simulink model "v_f_control_system"  (Simulink 8.9)
settings: Solver=ode23  StartTime=0.0  StopTime=5  RelTol=1e-3  EnableMultiTasking=on
undefined symbols (not defined in the file or in its folder): D1, Delta, DiscIntNeverNeededParam, Ts_Control, Ts_Power
libraries: powerlib x14, powerlib_meascontrol x9, simulink_extras x1, simulink x1
settings Model: Creator=Administrator  LastModifiedBy=Administrator
settings OptimizationCC: ExpressionDepthLimit=2147483647
settings DebuggingCC: SolverPrmCheckMsg=warning
settings GRTTargetCC: CombineOutputUpdateFcns=on  GRTInterface=off

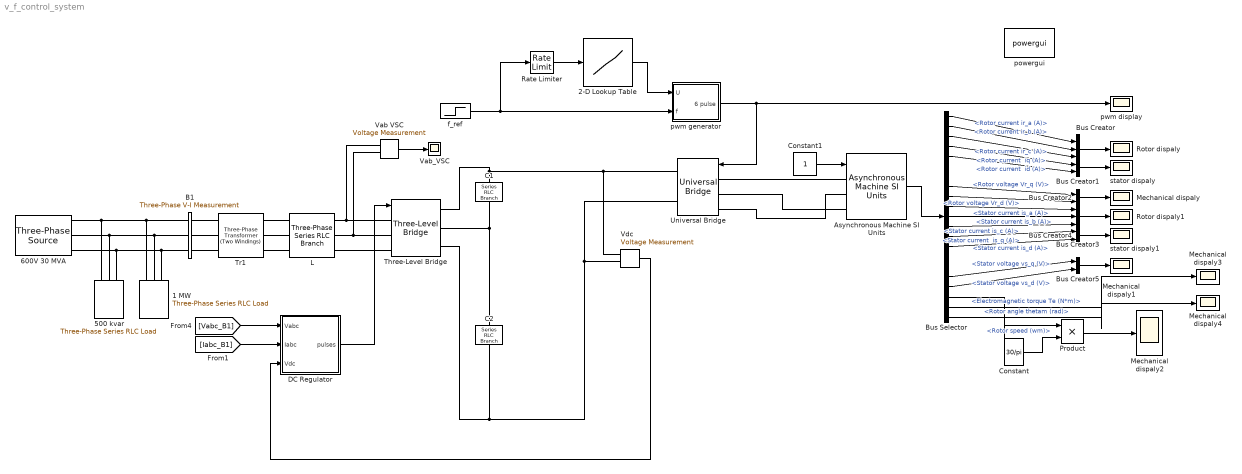
== system v_f_control_system ==
  1 MW : powerlib/Elements/Three-Phase Series RLC Load  LConnTagsString=A|B|C  Configuration=Y (grounded)  NominalVoltage=600  Vabc=[1e3 1e3 1e3]  Vabcp=[1e3 1e3 1e3]  NominalFrequency=60  UnbalancedPower=off  ActivePower=1e6  InductivePower=0  CapacitivePower=0  Pabc=[10e3 9e3 11e3]  QLabc=[100 90 110]  QCabc=[100 90 110]  Pabcp=[10e3 9e3 11e3]  QLabcp=[100 90 110]  QCabcp=[100 90 110]  Measurements=None  LoadType=constant Z
  2-D Lookup Table : Lookup_n-D  NumberOfTableDimensions=1  BreakpointsForDimension1=[0 5 25 50 100]  BreakpointsForDimension2=[1:3]  Table=[0.1 0.1 0.5 1 1]  RndMeth=Simplest  InputSameDT=on
  500 kvar : powerlib/Elements/Three-Phase Series RLC Load  LConnTagsString=A|B|C  Configuration=Y (grounded)  NominalVoltage=600  Vabc=[1e3 1e3 1e3]  Vabcp=[1e3 1e3 1e3]  NominalFrequency=60  UnbalancedPower=off  ActivePower=0.5e6/100  InductivePower=0  CapacitivePower=0.5e6  Pabc=[10e3 9e3 11e3]  QLabc=[100 90 110]  QCabc=[100 90 110]  Pabcp=[10e3 9e3 11e3]  QLabcp=[100 90 110]  QCabcp=[100 90 110]  Measurements=None  LoadType=constant Z
  600V 30 MVA : powerlib/Electrical Sources/Three-Phase Source  InternalConnection=Yg  VoltagePhases=off  Voltage=110  PhaseAngle=0  Voltage_phases=[25e3 25e3 25e3]/sqrt(3)  PhaseAngles_phases=[0 -120 +120]  Frequency=60  NonIdealSource=on  SpecifyImpedance=on  Resistance=0.724  Inductance=19.2e-3  ShortCircuitLevel=30e6  BaseVoltage=600  XRratio=10  BusType=swing  Pref=0  Qref=0  Prefabc=[10e3, 10e3, 10e3]  Qrefabc=[0, 0, 0]  Qmin=-inf  Qmax=inf
  Asynchronous Machine SI Units : powerlib/Machines/Asynchronous Machine SI Units  RotorType=Squirrel-cage  PresetModel=No  MechanicalLoad=Torque Tm  ShowDetailedParameters=on  ReferenceFrame=Rotor  Units=SI  MeasurementBus=off  NominalParameters=[ 2200, 380, 50 ]  Stator=[ 3.478 0.01254]  Rotor=[ 2.546 0.01226]  Cage1=[ 0.022 0.226/377]  Cage2=[ 0.022 0.226/377]  Lm=0.3329  Mechanical="[ 0.0131  0  2 ]"  PolePairs=2  InitialConditions=[1 0 0 0 0 0 0 0]  SimulateSaturation=off  Saturation=[14.03593122, 27.81365428, 53.79336849, 72.68890987, 97.98006896, 148.6815601, 215.7428561, 302.9841135, 420.4778367 ; 230, 322, 414, 460, 506, 552, 598, 644, 690]  LoadFlowParameters=1492000  TsPowergui=0  TsBlock=-1  IterativeModel=Forward Euler  IterativeDiscreteModel=Trapezoidal non iterative  Pmec=0
  B1 : powerlib/Measurements/Three-Phase V-I Measurement  VoltageMeasurement=phase-to-ground  SetLabelV=on  LabelV=Vabc_B1  Vpu=off  VpuLL=off  CurrentMeasurement=yes  SetLabelI=on  LabelI=Iabc_B1  Ipu=off  Pbase=100e6  Vbase=500e3  OutputType=Magnitude  PhasorSimulation=off  PSBequivalent=0
  Bus Creator : BusCreator  Inputs=3
  Bus Creator{1..2,4..5} (4 alike) : BusCreator  Inputs=2
  Bus Creator3 : BusCreator  Inputs=3
  Bus Selector : BusSelector  OutputSignals="Rotor measurements.Rotor current ir_a (A),Rotor measurements.Rotor current ir_b (A),Rotor measurements.Rotor current ir_c (A),Rotor measurements.Rotor current  iq (A),Rotor measurements.Rotor current  id (A),Rotor measurements.Rotor flux phir_q (V s),Rotor measurements.Rotor flux phir_d (V s),Rotor measurements.Rotor voltage Vr_q (V),Rotor measurements.Rotor voltage Vr_d (V),Stator measurements.Stator current is_a (A),Stator measurements.Stator current is_b (A),Stator measurements.Stator current is_c (A),Stator measurements.Stator current  is_q (A),Stator measurements.Stator current is_d (A),Stator measurements.Stator flux phis_q (V s),Stator measurements.Stator flux phis_d (V s),Stator measurements.Stator voltage vs_q (V),Stator measurements.Stator voltage vs_d (V),Mechanical.Rotor speed (wm),Mechanical.Electromagnetic torque Te (N*m),Mechanical.Rotor angle thetam (rad)"
  C1 : powerlib/Elements/Series RLC Branch  LConnTagsString=__new0  RConnTagsString=__new0  BranchType=C  Resistance=1.0  Inductance=1.0  SetiL0=off  InitialCurrent=0  Capacitance=0.1  Setx0=off  InitialVoltage=0  Measurements=None
  C2 : powerlib/Elements/Series RLC Branch  LConnTagsString=__new0  RConnTagsString=__new0  BranchType=C  Resistance=1.0  Inductance=1.0  SetiL0=off  InitialCurrent=0  Capacitance=0.1  Setx0=off  InitialVoltage=0  Measurements=None
  Constant : Constant  Value=30/pi
  Constant1 : Constant
  DC Regulator : Subsystem  mask(DC Voltage Regulator){Vdc_Ref=155.56}
      mask prompts: Vdc_Ref "DC voltage setpoint (V):"
  L : powerlib/Elements/Three-Phase Series RLC Branch  LConnTagsString=A|B|C  RConnTagsString=A|B|C  BranchType=RL  Resistance=0.1e-3  Inductance=20e-6  Capacitance=inf  Measurements=None
  Mechanical dispaly{,1..4} (5 alike) : Scope
  Product : Product
  Rate Limiter : RateLimiter  RisingSlewLimit=200  FallingSlewLimit=-200
  Rotor dispaly : Scope
  Rotor dispaly1 : Scope
  Three-Level Bridge : powerlib/Power Electronics/Three-Level Bridge  Arms=3  SnubberResistance=50  SbubberCapacitance=1e-6  Device=IGBT / Diodes  Ron=0.2e-3  ForwardVoltages="[  2 1 ]"  Measurements=All voltages and currents
      settings: SourceProductName=Simscape Power Systems  SourceProductBaseCode=PS
  Tr1 : powerlib/Elements/Three-Phase Transformer (Two Windings)  Winding1Connection=Yg  Winding2Connection=Delta (D1)  CoreType=Three single-phase transformers  SetSaturation=off  Hysteresis=off  DataFile='hysteresis'  SetInitialFlux=off  Measurements=None  UNITS=pu  NominalPower=[ 500e3 , 60 ]  Winding1=[ 110 , 0.04/30/2 , 0.04 ]  Winding2=[ 80 , 0.04/30/2 , 0.0 ]  Rm=500  Lm=500  L0=0.5  Saturation=[ 0,0 ; 0.0024,1.2 ; 1.0,1.52 ]  InitialFluxes=[ 0.8 , -0.8 , 0.7 ]  MoreParameters=off  BreakLoop=off  DataType=off  TransfoNumber=0
  Universal Bridge : powerlib/Power Electronics/Universal Bridge  Arms=3  SnubberResistance=1e5  SnubberCapacitance=inf  Device=IGBT / Diodes  Ron=1e-3  Lon=0  ForwardVoltages="[  0  0  ]"  ForwardVoltage=0  GTOparameters=[ 10e-6 , 20e-6 ]  IGBTparameters=[ 1e-6 , 2e-6 ]  Measurements=None  Measurements_2=None  converterType=Rectifier
  Vab VSC : powerlib/Measurements/Voltage Measurement  Tag=PoWeRsYsTeMmEaSuReMeNt  PhasorSimulation=off  OutputType=Magnitude  PSBequivalent=0
  Vab_VSC : Scope
  "Vdc " : powerlib/Measurements/Voltage Measurement  Tag=PoWeRsYsTeMmEaSuReMeNt  PhasorSimulation=off  OutputType=Magnitude  PSBequivalent=0
  f_ref : Step  Time=100  Before=33  After=33  SampleTime=0
  powergui : powerlib/powergui  Priority=1  SimulationMode=Discrete  SampleTime=1e-5  frequency=60  Iterations=50  frequencyindice=50  Pbase=100e6  ErrMax=1e-4  UnitsV=kV  UnitsW=MW  buscounter=0  FunctionMessages=off  echomessages=off  EnableUseOfTLC=off  CurrentSourceSwitches=off  DisableSnubberDevices=off  DisableRonSwitches=off  DisableVfSwitches=off  DisplayEquations=off  SolverType=Tustin  Interpol=off  ExternalGateDelay=off  methode=off  Ts=100  x0status=blocks  SPID=off  SwTol=0  HookPort=off  RestoreLinks=warning  ResistiveCurrentMeasurement=off  Frange=[0:2:500]  Ylog=off  Xlog=on  ShowGrid=off  save=off  variable=ZData  structure=0  ZoomFFT=off  StartTime=0.0  cycles=1  DisplayStyle=1  fundamental=60  FreqAxis=off  MaxFrequency=1000  frequencyindicesteady=1  RmsSteady=1  display=off
  pwm display : Scope
  pwm generator : Subsystem
  stator dispaly : Scope
  stator dispaly1 : Scope
  wires:
  pwm generator/1(6 pulse) -> Universal Bridge/1, pwm display/1
  f_ref/1 -> pwm generator/2(f), Rate Limiter/1
  Rate Limiter/1 -> 2-D Lookup Table/1
  2-D Lookup Table/1 -> pwm generator/1(U)
  Constant1/1 -> Asynchronous Machine SI Units/1
  Asynchronous Machine SI Units/1 -> Bus Selector/1
  Bus Selector/1 -> Bus Creator/1  "<Rotor current ir_a (A)>"
  Bus Selector/2 -> Bus Creator/2  "<Rotor current ir_b (A)>"
  Bus Selector/3 -> Bus Creator/3  "<Rotor current ir_c (A)>"
  Bus Creator/1 -> Rotor dispaly/1
  Bus Selector/4 -> Bus Creator1/1  "<Rotor current  iq (A)>"
  Bus Selector/5 -> Bus Creator1/2  "<Rotor current  id (A)>"
  Bus Selector/8 -> Bus Creator2/1  "<Rotor voltage Vr_q (V)>"
  Bus Selector/9 -> Bus Creator2/2  "<Rotor voltage Vr_d (V)>"
  Bus Creator1/1 -> stator dispaly/1
  Bus Creator2/1 -> Mechanical dispaly/1
  Bus Creator3/1 -> Rotor dispaly1/1
  Bus Creator4/1 -> stator dispaly1/1
  Bus Creator5/1 -> Mechanical dispaly1/1
  Bus Selector/10 -> Bus Creator3/1  "<Stator current is_a (A)>"
  Bus Selector/11 -> Bus Creator3/2  "<Stator current is_b (A)>"
  Bus Selector/12 -> Bus Creator3/3  "<Stator current is_c (A)>"
  Bus Selector/13 -> Bus Creator4/1  "<Stator current  is_q (A)>"
  Bus Selector/14 -> Bus Creator4/2  "<Stator current is_d (A)>"
  Bus Selector/17 -> Bus Creator5/1  "<Stator voltage vs_q (V)>"
  Bus Selector/18 -> Bus Creator5/2  "<Stator voltage vs_d (V)>"
  Bus Selector/20 -> Mechanical dispaly3/1  "<Electromagnetic torque Te (N*m)>"
  Bus Selector/21 -> Mechanical dispaly4/1  "<Rotor angle thetam (rad)>"
  Bus Selector/19 -> Product/1  "<Rotor speed (wm)>"
  Constant/1 -> Product/2
  Product/1 -> Mechanical dispaly2/1
  Vab VSC/1 -> Vab_VSC/1
  [Iabc_B1] -> DC Regulator/2(Iabc)
  "Vdc "/1 -> DC Regulator/3(Vdc)
  [Vabc_B1] -> DC Regulator/1(Vabc)
  DC Regulator/1(pulses) -> Three-Level Bridge/1
  connections:
  Universal Bridge/LConn1 -- Asynchronous Machine SI Units/LConn1
  C1/LConn1 -- Three-Level Bridge/RConn1 -- "Vdc "/LConn1 -- Universal Bridge/RConn1
  1 MW/LConn1 -- B1/LConn1 -- 500 kvar/LConn1 -- 600V 30 MVA/RConn1
  C1/RConn1 -- Three-Level Bridge/RConn2 -- C2/LConn1
  Three-Level Bridge/LConn2 -- Vab VSC/LConn2 -- L/RConn2
  1 MW/LConn3 -- B1/LConn3 -- 500 kvar/LConn3 -- 600V 30 MVA/RConn3
  1 MW/LConn2 -- B1/LConn2 -- 500 kvar/LConn2 -- 600V 30 MVA/RConn2
  Three-Level Bridge/LConn1 -- Vab VSC/LConn1 -- L/RConn1
  C2/RConn1 -- "Vdc "/LConn2 -- Universal Bridge/RConn2 -- Three-Level Bridge/RConn3
  Tr1/RConn1 -- L/LConn1
  B1/RConn2 -- Tr1/LConn2
  Tr1/RConn3 -- L/LConn3
  B1/RConn1 -- Tr1/LConn1
  B1/RConn3 -- Tr1/LConn3
  Tr1/RConn2 -- L/LConn2
  L/RConn3 -- Three-Level Bridge/LConn3
  Universal Bridge/LConn2 -- Asynchronous Machine SI Units/LConn3
  Universal Bridge/LConn3 -- Asynchronous Machine SI Units/LConn2

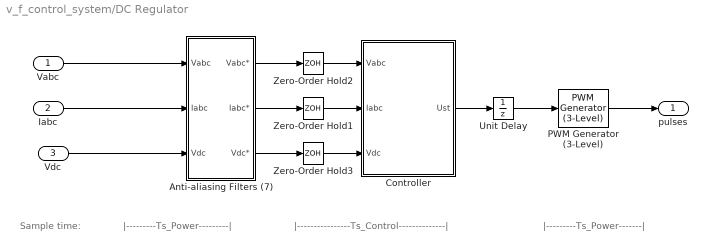
== system v_f_control_system/DC Regulator ==
  note: |----------------Ts_Control--------------|
  note: |---------Ts_Power---------|
  note: Sample time:
  note: |---------Ts_Power-------|
  Vabc : Inport  PortDimensions=3
  Iabc : Inport  Port=2  PortDimensions=3
  Vdc : Inport  Port=3  PortDimensions=1
  Anti-aliasing Filters (7) : Subsystem  mask(Anti-aliasing (2nd order lowpass)){Fc=750, Ts=Ts_Power}
      mask prompts: Fc "Cut-off frequency (Hz):"; Ts "Sample time:"
  Controller : Subsystem  mask(DC Regulator){Vdc_Ref=Vdc_Ref, Par_VdcReg=[0.015 1.6], Par_IReg=[0.3 20], Par_Nom=[600 500e3], Ts=Ts_Control}
      mask prompts: Vdc_Ref "DC Voltage setpoint (Volts)"; Par_VdcReg "Vdc Regulator Gains: [ Kp  Ki ]"; Par_IReg "Current Regulators Gain: [ Kp Ki Kd ]"; Par_Nom "Nominal Voltage and power: [ Vnom (volts rms L-L)  Pnom (VA) ]"; Ts "Time Step (s)"
      mask init:
      | Vnom=Par_Nom(1);
      | Pnom=Par_Nom(2);
      | Kp_I=Par_IReg(1);
      | Ki_I=Par_IReg(2);
      | Kp_Vdc=Par_VdcReg(1);
      | Ki_Vdc=Par_VdcReg(2);
  PWM Generator (3-Level) : powerlib_meascontrol/Pulse & Signal Generators/PWM Generator (3-Level)  ModulatorType=Three-phase bridge (12 pulses)  ModulatorMode=Unsynchronized  nF=27  Fc=27*60  ModulatingSignals=off  m=0.8  Freq=60  Phase=0  Ts=Ts_Power
      settings: SourceProductName=Simscape Power Systems  SourceProductBaseCode=PS
  Unit Delay : UnitDelay  SampleTime=Ts_Control
  Zero-Order Hold1 : ZeroOrderHold  SampleTime=Ts_Control
  Zero-Order Hold2 : ZeroOrderHold  SampleTime=Ts_Control
  Zero-Order Hold3 : ZeroOrderHold  SampleTime=Ts_Control
  pulses : Outport
  wires:
  PWM Generator (3-Level)/1 -> pulses/1
  Unit Delay/1 -> PWM Generator (3-Level)/1
  Controller/1(Ust) -> Unit Delay/1
  Anti-aliasing Filters (7)/1(" Vabc*") -> Zero-Order Hold2/1
  Anti-aliasing Filters (7)/2(Iabc*) -> Zero-Order Hold1/1
  Anti-aliasing Filters (7)/3(" Vdc*") -> Zero-Order Hold3/1
  Zero-Order Hold3/1 -> Controller/3(Vdc)
  Zero-Order Hold1/1 -> Controller/2(Iabc)
  Zero-Order Hold2/1 -> Controller/1(Vabc)
  Vdc/1 -> Anti-aliasing Filters (7)/3("Vdc ")
  Iabc/1 -> Anti-aliasing Filters (7)/2("Iabc ")
  Vabc/1 -> Anti-aliasing Filters (7)/1(Vabc)

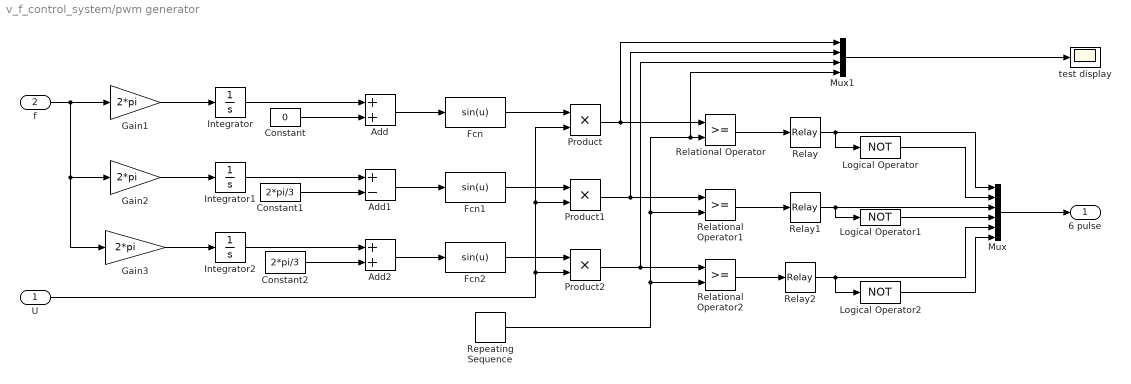
== system v_f_control_system/pwm generator ==
  U : Inport
  f : Inport  Port=2
  Add : Sum
  Add1 : Sum  Inputs=+-
  Add2 : Sum
  Constant : Constant  Value=0
  Constant1 : Constant  Value=2*pi/3
  Constant2 : Constant  Value=2*pi/3
  Fcn : Fcn  Expr=sin(u)
  Fcn1 : Fcn  Expr=sin(u)
  Fcn2 : Fcn  Expr=sin(u)
  Gain1 : Gain  Gain=2*pi
  Gain2 : Gain  Gain=2*pi
  Gain3 : Gain  Gain=2*pi
  Integrator : Integrator
  Integrator1 : Integrator
  Integrator2 : Integrator
  Logical Operator : Logic  Operator=NOT  AllPortsSameDT=off  OutDataTypeStr=boolean
  Logical Operator1 : Logic  Operator=NOT  AllPortsSameDT=off  OutDataTypeStr=boolean
  Logical Operator2 : Logic  Operator=NOT  AllPortsSameDT=off  OutDataTypeStr=boolean
  Mux : Mux  Inputs=6
  Mux1 : Mux
  Product : Product  RndMeth=Zero
  Product1 : Product  RndMeth=Zero
  Product2 : Product  RndMeth=Zero
  Relational Operator : RelationalOperator  OutDataTypeStr=boolean  RndMeth=Nearest
  Relational Operator1 : RelationalOperator  OutDataTypeStr=boolean  RndMeth=Nearest
  Relational Operator2 : RelationalOperator  OutDataTypeStr=boolean  RndMeth=Nearest
  Relay : Relay
  Relay1 : Relay
  Relay2 : Relay
  Repeating Sequence : simulink/Sources/Repeating Sequence  rep_seq_t=[0 0.5/3000 1/3000]  rep_seq_y=[-1 1 -1]
  test display : Scope
  6 pulse : Outport
  wires:
  f/1 -> Gain1/1, Gain3/1, Gain2/1
  Gain1/1 -> Integrator/1
  Gain2/1 -> Integrator1/1
  Gain3/1 -> Integrator2/1
  Integrator/1 -> Add/1
  Integrator1/1 -> Add1/1
  Integrator2/1 -> Add2/1
  Constant/1 -> Add/2
  Constant1/1 -> Add1/2
  Constant2/1 -> Add2/2
  Add/1 -> Fcn/1
  Add1/1 -> Fcn1/1
  Add2/1 -> Fcn2/1
  Repeating Sequence/1 -> Relational Operator2/2, Relational Operator1/2, Relational Operator/2, Mux1/4
  Relational Operator/1 -> Relay/1
  Relational Operator1/1 -> Relay1/1
  Relational Operator2/1 -> Relay2/1
  Mux/1 -> 6 pulse/1
  Fcn/1 -> Product/1
  Fcn2/1 -> Product2/1
  Fcn1/1 -> Product1/1
  U/1 -> Product1/2, Product/2, Product2/2
  Product/1 -> Relational Operator/1, Mux1/1
  Product2/1 -> Relational Operator2/1, Mux1/3
  Product1/1 -> Relational Operator1/1, Mux1/2
  Relay/1 -> Mux/1, Logical Operator/1
  Logical Operator/1 -> Mux/2
  Relay1/1 -> Mux/3, Logical Operator1/1
  Logical Operator1/1 -> Mux/4
  Relay2/1 -> Mux/5, Logical Operator2/1
  Logical Operator2/1 -> Mux/6
  Mux1/1 -> test display/1

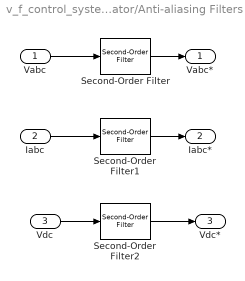
== system v_f_control_system/DC Regulator/Anti-aliasing Filters (7) ==
  Vabc : Inport  PortDimensions=3
  "Iabc " : Inport  Port=2  PortDimensions=3
  "Vdc " : Inport  Port=3  PortDimensions=1
  Second-Order Filter : powerlib_meascontrol/Filters/Second-Order Filter  FilterType=Lowpass  Fo=Fc  Zeta=0.707  Ts=Ts  Initialize=off  Vac_Init="[0,  0,  60]"  Vdc_Init=0  PlotResponse=off  FreqRange=[0, 500, 1]
      settings: SourceProductName=Simscape Power Systems  SourceProductBaseCode=PS
  Second-Order Filter1 : powerlib_meascontrol/Filters/Second-Order Filter  FilterType=Lowpass  Fo=Fc  Zeta=0.707  Ts=Ts  Initialize=off  Vac_Init="[0,  0,  60]"  Vdc_Init=0  PlotResponse=off  FreqRange=[0, 500, 1]
      settings: SourceProductName=Simscape Power Systems  SourceProductBaseCode=PS
  Second-Order Filter2 : powerlib_meascontrol/Filters/Second-Order Filter  FilterType=Lowpass  Fo=Fc  Zeta=0.707  Ts=Ts  Initialize=off  Vac_Init="[0,  0,  60]"  Vdc_Init=0  PlotResponse=off  FreqRange=[0, 500, 1]
      settings: SourceProductName=Simscape Power Systems  SourceProductBaseCode=PS
  " Vabc*" : Outport
  Iabc* : Outport  Port=2
  " Vdc*" : Outport  Port=3
  wires:
  Second-Order Filter2/1 -> " Vdc*"/1
  "Vdc "/1 -> Second-Order Filter2/1
  Vabc/1 -> Second-Order Filter/1
  Second-Order Filter/1 -> " Vabc*"/1
  "Iabc "/1 -> Second-Order Filter1/1
  Second-Order Filter1/1 -> Iabc*/1

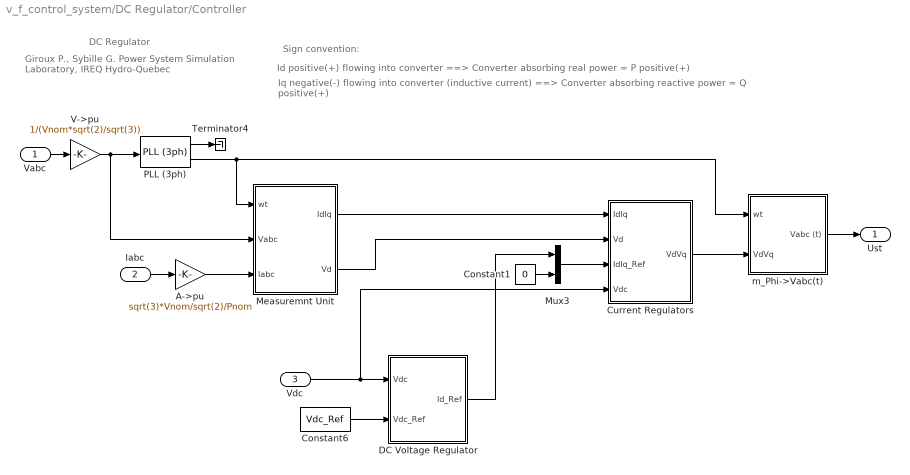
== system v_f_control_system/DC Regulator/Controller ==
  note: DC Regulator
  note: Giroux P., Sybille G.
      | Power System Simulation Laboratory, IREQ
      | Hydro-Quebec
  note: Iq negative(-) flowing into converter (inductive current) ==> Converter absorbing reactive power = Q positive(+)
  note: Sign convention:
  note: Id positive(+) flowing into converter ==> Converter absorbing real power = P positive(+)
  Vabc : Inport  PortDimensions=3
  Iabc : Inport  Port=2  PortDimensions=3
  Vdc : Inport  Port=3  PortDimensions=1
  A->pu : Gain  Gain=sqrt(3)*Vnom/sqrt(2)/Pnom  SaturateOnIntegerOverflow=on  OutDataTypeStr=Inherit: Same as input  ParamDataTypeStr=Inherit: Same as input
  Constant1 : Constant  Value=0
  Constant6 : Constant  Value=Vdc_Ref
  Current Regulators : Subsystem  mask(Current Regulators){Kp=Kp_I, Ki=Ki_I, Kd=0, TcD=0.2e-3, Par_Limits=[12 -12], Init=0, Ts=Ts}
      mask prompts: Kp "Proportional gain (Kp):"; Ki "Integral gain (Ki):"; Kd "Derivative gain (Kd):"; TcD "Time constant for derivative (s):"; Par_Limits "Output limits: [ Upper   Lower ]"; Init "Output initial value:"; Ts "Sample time:"
      mask help:
      | Sign convention:
      | Id positive(+) flowing into converter ==> Converter absorbing real power = P positive(+)
      | Iq negative(-) flowing into converter (inductive current) ==> Converter absorbing reactive power = Q positive(+)
  DC Voltage Regulator : Subsystem  mask(DC Voltage regulator){Kp=Kp_Vdc, Ki=Ki_Vdc, Ts=Ts}
      mask prompts: Kp "Proportional gain (Kp):"; Ki "Integral gain(Ki)"; Ts "Sample time:"
  Measuremnt Unit : Subsystem
  Mux3 : Mux  Inputs=2
  PLL (3ph) : powerlib_meascontrol/PLL/PLL (3ph)  Fmin=45  Par_Init=[-45 60]  ParK=[60 1400]  TcD=1e-4  MaxRateChangeFreq=12  FilterCutOffFreq=25  Ts=Ts  AGC=off
  Terminator4 : Terminator
  V->pu : Gain  Gain=1/(Vnom*sqrt(2)/sqrt(3))  SaturateOnIntegerOverflow=on  OutDataTypeStr=Inherit: Same as input  ParamDataTypeStr=Inherit: Same as input
  m_Phi->Vabc(t) : Subsystem
  Ust : Outport
  wires:
  m_Phi->Vabc(t)/1(Vabc (t)) -> Ust/1
  PLL (3ph)/2 -> m_Phi->Vabc(t)/1(wt), Measuremnt Unit/1(wt)
  Current Regulators/1(VdVq) -> m_Phi->Vabc(t)/2(VdVq)
  DC Voltage Regulator/1(Id_Ref) -> Mux3/1
  Constant1/1 -> Mux3/2
  Mux3/1 -> Current Regulators/3(IdIq_Ref)
  Measuremnt Unit/2(Vd) -> Current Regulators/2(Vd)
  Measuremnt Unit/1(IdIq) -> Current Regulators/1(IdIq)
  Iabc/1 -> A->pu/1
  PLL (3ph)/1 -> Terminator4/1
  Vdc/1 -> Current Regulators/4(Vdc), DC Voltage Regulator/1(Vdc)
  Constant6/1 -> DC Voltage Regulator/2(Vdc_Ref)
  Vabc/1 -> V->pu/1
  V->pu/1 -> PLL (3ph)/1, Measuremnt Unit/2(Vabc)
  A->pu/1 -> Measuremnt Unit/3(Iabc)

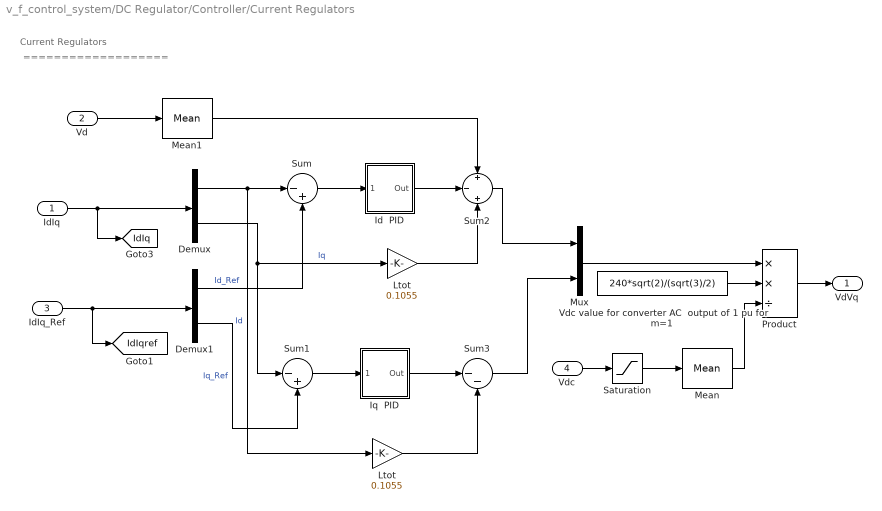
== system v_f_control_system/DC Regulator/Controller/Current Regulators ==
  note: ===================
  note: Current Regulators
  IdIq : Inport  PortDimensions=2
  Vd : Inport  Port=2
  IdIq_Ref : Inport  Port=3  PortDimensions=2
  Vdc : Inport  Port=4
  " Ltot" : Gain  Gain=0.1055  SaturateOnIntegerOverflow=on  OutDataTypeStr=Inherit: Same as input  ParamDataTypeStr=Inherit: Same as input
  Demux : Demux  Outputs=2
  Demux1 : Demux  Outputs=2
  Id  PID : Subsystem  DialogController=POWERSYS.PowerSysDialog  mask(Discrete PID Controller){Kp=Kp, Ki=Ki, Kd=Kd, TcD=TcD, Par_Limits=Par_Limits, Init=Init, Ts=Ts}
      mask prompts: Kp "Proportional gain (Kp):"; Ki "Integral gain (Ki):"; Kd "Derivative gain (Kd):"; TcD "Time constant for derivative (s):"; Par_Limits "Output limits: [ Upper   Lower ]"; Init "Output initial value:"; Ts "Sample time:"
      mask help: This block implements a discrete PID controller.
      mask init:
      | UpperLimit=Par_Limits(1);
      | LowerLimit=Par_Limits(2);
      | power_initmask();
      mask Display: disp('PID');
  Iq  PID : Subsystem  DialogController=POWERSYS.PowerSysDialog  mask(Discrete PID Controller){Kp=Kp, Ki=Ki, Kd=Kd, TcD=TcD, Par_Limits=Par_Limits, Init=Init, Ts=Ts}
      mask prompts: Kp "Proportional gain (Kp):"; Ki "Integral gain (Ki):"; Kd "Derivative gain (Kd):"; TcD "Time constant for derivative (s):"; Par_Limits "Output limits: [ Upper   Lower ]"; Init "Output initial value:"; Ts "Sample time:"
      mask help: This block implements a discrete PID controller.
      mask init:
      | UpperLimit=Par_Limits(1);
      | LowerLimit=Par_Limits(2);
      | power_initmask();
      mask Display: disp('PID');
  "Ltot " : Gain  Gain=0.1055  SaturateOnIntegerOverflow=on  OutDataTypeStr=Inherit: Same as input  ParamDataTypeStr=Inherit: Same as input
  Mean : powerlib_meascontrol/Measurements/Mean  Freq=60  Vinit=500  Ts=Ts
  Mean1 : powerlib_meascontrol/Measurements/Mean  Freq=60  Vinit=1.007  Ts=Ts
  Mux : Mux  Inputs=2
  Product : Product  Inputs=**/  SaturateOnIntegerOverflow=on  InputSameDT=on  OutDataTypeStr=Inherit: Same as first input
  Saturation : Saturate  UpperLimit=10000  LowerLimit=10
  Sum : Sum  Inputs=|-+  SaturateOnIntegerOverflow=on  InputSameDT=on  OutDataTypeStr=Inherit: Same as first input
  Sum1 : Sum  Inputs=|-+  SaturateOnIntegerOverflow=on  InputSameDT=on  OutDataTypeStr=Inherit: Same as first input
  Sum2 : Sum  Inputs=+|-|+  SaturateOnIntegerOverflow=on  InputSameDT=on  OutDataTypeStr=Inherit: Same as first input
  Sum3 : Sum  Inputs=|--  SaturateOnIntegerOverflow=on  InputSameDT=on  OutDataTypeStr=Inherit: Same as first input
  Vdc value for converter AC  output of 1 pu for m=1 : Constant  Value=240*sqrt(2)/(sqrt(3)/2)
  VdVq : Outport
  tag scope: IdIq=global, IdIqref=global
  wires:
  Sum3/1 -> Mux/2
  Vdc/1 -> Saturation/1
  Mean/1 -> Product/3
  Vdc value for converter AC  output of 1 pu for m=1/1 -> Product/2
  Saturation/1 -> Mean/1
  Mean1/1 -> Sum2/1
  Product/1 -> VdVq/1
  IdIq_Ref/1 -> [IdIqref], Demux1/1
  Mux/1 -> Product/1
  Sum/1 -> Id  PID/1(Error)
  Demux1/2 -> Sum1/2  "Iq_Ref"
  Sum1/1 -> Iq  PID/1(Error)
  Demux/2 -> Sum1/1, "Ltot "/1  "Iq"
  Demux1/1 -> Sum/2  "Id_Ref"
  Demux/1 -> " Ltot"/1, Sum/1  "Id"
  IdIq/1 -> [IdIq], Demux/1
  Id  PID/1(Out) -> Sum2/2
  Sum2/1 -> Mux/1
  Iq  PID/1(Out) -> Sum3/1
  "Ltot "/1 -> Sum2/3
  " Ltot"/1 -> Sum3/2
  Vd/1 -> Mean1/1

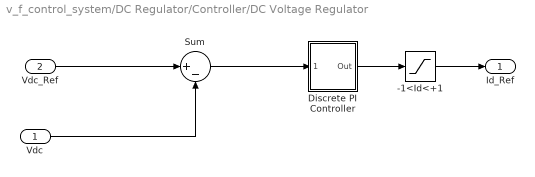
== system v_f_control_system/DC Regulator/Controller/DC Voltage Regulator ==
  Vdc : Inport
  Vdc_Ref : Inport  Port=2
  -1<Id<+1 : Saturate  UpperLimit=1.2  LowerLimit=-1.2
  Discrete PI Controller : Subsystem  DialogController=POWERSYS.PowerSysDialog  mask(Discrete PI Controller){Kp=Kp, Ki=Ki, Par_Limits=[1.2 -1.2], Init=0, Ts=Ts}
      mask prompts: Kp "Proportional gain (Kp):"; Ki "Integral gain (Ki):"; Par_Limits "Output limits: [ Upper   Lower ]"; Init "Output initial value:"; Ts "Sample time:"
      mask help: This block implements a discrete PI controller.
      mask init:
      | UpperLimit=Par_Limits(1);
      | LowerLimit=Par_Limits(2);
      | power_initmask();
      mask Display: disp('PI');
  Sum : Sum  Inputs=|+-  SaturateOnIntegerOverflow=on  InputSameDT=on  OutDataTypeStr=Inherit: Same as first input
  Id_Ref : Outport  InitialOutput=0
  wires:
  Sum/1 -> Discrete PI Controller/1(Error)
  Vdc/1 -> Sum/2
  Discrete PI Controller/1(Out) -> -1<Id<+1/1
  -1<Id<+1/1 -> Id_Ref/1
  Vdc_Ref/1 -> Sum/1

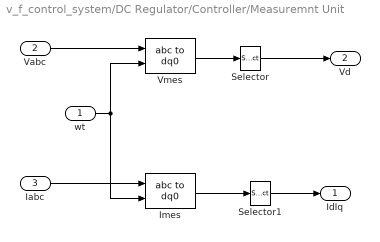
== system v_f_control_system/DC Regulator/Controller/Measuremnt Unit ==
  wt : Inport
  Vabc : Inport  Port=2
  Iabc : Inport  Port=3
  Imes : powerlib_meascontrol/Transformations/abc to dq0  Alignment=90 degrees behind phase A axis
  Selector : Selector  InputPortWidth=3  IndexOptions=Index vector (dialog)  Indices=1  OutputSizes=1
  Selector1 : Selector  InputPortWidth=3  IndexOptions=Index vector (dialog)  Indices=[1 2]  OutputSizes=1
  Vmes : powerlib_meascontrol/Transformations/abc to dq0  Alignment=90 degrees behind phase A axis
  IdIq : Outport
  Vd : Outport  Port=2
  wires:
  Selector/1 -> Vd/1
  Imes/1 -> Selector1/1
  Iabc/1 -> Imes/1
  wt/1 -> Imes/2, Vmes/2
  Vmes/1 -> Selector/1
  Vabc/1 -> Vmes/1
  Selector1/1 -> IdIq/1

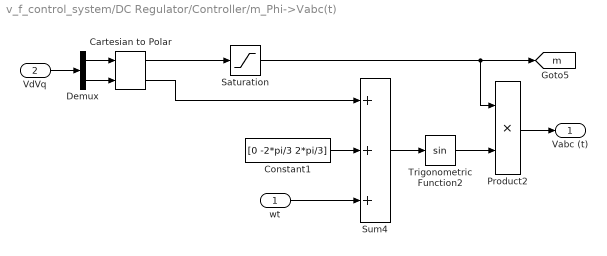
== system v_f_control_system/DC Regulator/Controller/m_Phi->Vabc(t) ==
  wt : Inport
  VdVq : Inport  Port=2
  Cartesian to Polar : simulink_extras/Transformations/Cartesian to Polar
      settings: SourceProductName=Simulink Extras
  Constant1 : Constant  Value=[0 -2*pi/3 2*pi/3]
  Demux : Demux  Outputs=2
  Product2 : Product  SaturateOnIntegerOverflow=on  InputSameDT=on  OutDataTypeStr=Inherit: Same as first input
  Saturation : Saturate  UpperLimit=1  LowerLimit=0
  Sum4 : Sum  Inputs=+++  SaturateOnIntegerOverflow=on  InputSameDT=on  OutDataTypeStr=Inherit: Same as first input
  Trigonometric Function2 : Trigonometry
  Vabc (t) : Outport
  tag scope: m=global
  wires:
  Saturation/1 -> [m], Product2/1
  Cartesian to Polar/1 -> Saturation/1
  Trigonometric Function2/1 -> Product2/2
  Sum4/1 -> Trigonometric Function2/1
  Cartesian to Polar/2 -> Sum4/1
  Demux/2 -> Cartesian to Polar/2
  Demux/1 -> Cartesian to Polar/1
  VdVq/1 -> Demux/1
  wt/1 -> Sum4/3
  Product2/1 -> Vabc (t)/1
  Constant1/1 -> Sum4/2

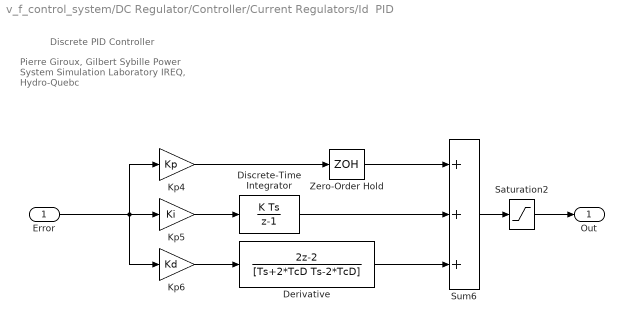
== system v_f_control_system/DC Regulator/Controller/Current Regulators/Id  PID ==
  note: Pierre Giroux, Gilbert Sybille
      | Power System Simulation Laboratory
      | IREQ, Hydro-Quebc
  note: Discrete PID Controller
  Error : Inport  SampleTime=Ts
  "Derivative " : DiscreteTransferFcn  Numerator=[2 -2]  Denominator=[Ts+2*TcD Ts-2*TcD]  SampleTime=Ts
  Discrete-Time Integrator : DiscreteIntegrator  InitialCondition=Init  SampleTime=Ts  LimitOutput=on  UpperSaturationLimit=UpperLimit  LowerSaturationLimit=LowerLimit  ICPrevOutput=DiscIntNeverNeededParam  ICPrevScaledInput=DiscIntNeverNeededParam
  Kp4 : Gain  Gain=Kp  SampleTime=Ts  SaturateOnIntegerOverflow=on  OutDataTypeStr=Inherit: Same as input  ParamDataTypeStr=Inherit: Same as input
  Kp5 : Gain  Gain=Ki  SampleTime=Ts  SaturateOnIntegerOverflow=on  OutDataTypeStr=Inherit: Same as input  ParamDataTypeStr=Inherit: Same as input
  Kp6 : Gain  Gain=Kd  SampleTime=Ts  SaturateOnIntegerOverflow=on  OutDataTypeStr=Inherit: Same as input  ParamDataTypeStr=Inherit: Same as input
  Saturation2 : Saturate  UpperLimit=UpperLimit  LowerLimit=LowerLimit  SampleTime=Ts
  Sum6 : Sum  Inputs=+++  SampleTime=Ts  SaturateOnIntegerOverflow=on  InputSameDT=on  OutDataTypeStr=Inherit: Same as first input
  Zero-Order Hold : ZeroOrderHold  SampleTime=Ts
  Out : Outport  SampleTime=Ts  InitialOutput=0
  wires:
  Saturation2/1 -> Out/1
  Error/1 -> Kp4/1, Kp5/1, Kp6/1
  Sum6/1 -> Saturation2/1
  Kp5/1 -> Discrete-Time Integrator/1
  Kp6/1 -> "Derivative "/1
  Kp4/1 -> Zero-Order Hold/1
  Discrete-Time Integrator/1 -> Sum6/2
  "Derivative "/1 -> Sum6/3
  Zero-Order Hold/1 -> Sum6/1

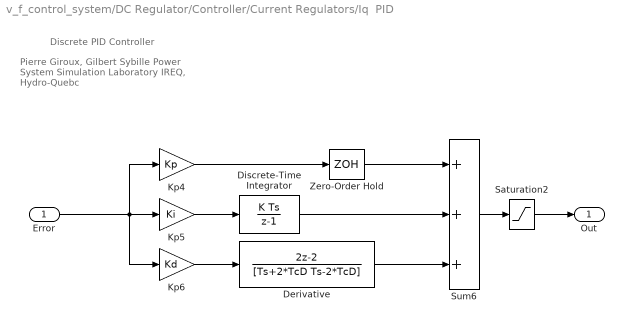
== system v_f_control_system/DC Regulator/Controller/Current Regulators/Iq  PID ==
  note: Pierre Giroux, Gilbert Sybille
      | Power System Simulation Laboratory
      | IREQ, Hydro-Quebc
  note: Discrete PID Controller
  Error : Inport  SampleTime=Ts
  "Derivative " : DiscreteTransferFcn  Numerator=[2 -2]  Denominator=[Ts+2*TcD Ts-2*TcD]  SampleTime=Ts
  Discrete-Time Integrator : DiscreteIntegrator  InitialCondition=Init  SampleTime=Ts  LimitOutput=on  UpperSaturationLimit=UpperLimit  LowerSaturationLimit=LowerLimit  ICPrevOutput=DiscIntNeverNeededParam  ICPrevScaledInput=DiscIntNeverNeededParam
  Kp4 : Gain  Gain=Kp  SampleTime=Ts  SaturateOnIntegerOverflow=on  OutDataTypeStr=Inherit: Same as input  ParamDataTypeStr=Inherit: Same as input
  Kp5 : Gain  Gain=Ki  SampleTime=Ts  SaturateOnIntegerOverflow=on  OutDataTypeStr=Inherit: Same as input  ParamDataTypeStr=Inherit: Same as input
  Kp6 : Gain  Gain=Kd  SampleTime=Ts  SaturateOnIntegerOverflow=on  OutDataTypeStr=Inherit: Same as input  ParamDataTypeStr=Inherit: Same as input
  Saturation2 : Saturate  UpperLimit=UpperLimit  LowerLimit=LowerLimit  SampleTime=Ts
  Sum6 : Sum  Inputs=+++  SampleTime=Ts  SaturateOnIntegerOverflow=on  InputSameDT=on  OutDataTypeStr=Inherit: Same as first input
  Zero-Order Hold : ZeroOrderHold  SampleTime=Ts
  Out : Outport  SampleTime=Ts  InitialOutput=0
  wires:
  Saturation2/1 -> Out/1
  Error/1 -> Kp4/1, Kp5/1, Kp6/1
  Sum6/1 -> Saturation2/1
  Kp5/1 -> Discrete-Time Integrator/1
  Kp6/1 -> "Derivative "/1
  Kp4/1 -> Zero-Order Hold/1
  Discrete-Time Integrator/1 -> Sum6/2
  "Derivative "/1 -> Sum6/3
  Zero-Order Hold/1 -> Sum6/1

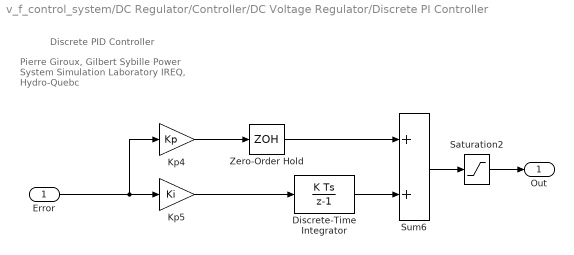
== system v_f_control_system/DC Regulator/Controller/DC Voltage Regulator/Discrete PI Controller ==
  note: Discrete PID Controller
  note: Pierre Giroux, Gilbert Sybille
      | Power System Simulation Laboratory
      | IREQ, Hydro-Quebc
  Error : Inport  SampleTime=Ts
  Discrete-Time Integrator : DiscreteIntegrator  InitialCondition=Init  SampleTime=Ts  LimitOutput=on  UpperSaturationLimit=UpperLimit  LowerSaturationLimit=LowerLimit  ICPrevOutput=DiscIntNeverNeededParam  ICPrevScaledInput=DiscIntNeverNeededParam
  Kp4 : Gain  Gain=Kp  SampleTime=Ts  SaturateOnIntegerOverflow=on  OutDataTypeStr=Inherit: Same as input  ParamDataTypeStr=Inherit: Same as input
  Kp5 : Gain  Gain=Ki  SampleTime=Ts  SaturateOnIntegerOverflow=on  OutDataTypeStr=Inherit: Same as input  ParamDataTypeStr=Inherit: Same as input
  Saturation2 : Saturate  UpperLimit=UpperLimit  LowerLimit=LowerLimit  SampleTime=Ts
  Sum6 : Sum  SampleTime=Ts  SaturateOnIntegerOverflow=on  InputSameDT=on  OutDataTypeStr=Inherit: Same as first input
  Zero-Order Hold : ZeroOrderHold  SampleTime=Ts
  Out : Outport  SampleTime=Ts  InitialOutput=0
  wires:
  Zero-Order Hold/1 -> Sum6/1
  Saturation2/1 -> Out/1
  Discrete-Time Integrator/1 -> Sum6/2
  Kp4/1 -> Zero-Order Hold/1
  Kp5/1 -> Discrete-Time Integrator/1
  Sum6/1 -> Saturation2/1
  Error/1 -> Kp5/1, Kp4/1
